simulink model "SBPAMemory"  (R2016a)
settings: Solver=VariableStepAuto  StartTime=0.0  StopTime=1  RelTol=1e-3
values from neighbouring files (symbols this model uses):
  Te = 0.001    [MatlabProjet.m]
libraries: simulink_extras x1
settings Model: Creator=luhernan  LastModifiedBy=luhernan

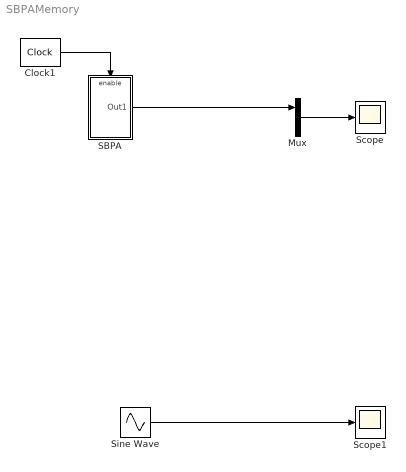
== system SBPAMemory ==
  Clock1 : simulink_extras/Flip Flops/Clock  period=PHorloge
  Mux : Mux  Inputs=2
  SBPA : Subsystem  mask{A=20, Offset=-10}
      mask prompts: A "gain"
  Scope : Scope
  Scope1 : Scope
  Sine Wave : Sin  Amplitude=10  Frequency=6*pi  SampleTime=Te
  wires:
  SBPA/1(Out1) -> Mux/1
  Clock1/1 -> SBPA/Enable
  Sine Wave/1 -> Scope1/1
  Mux/1 -> Scope/1

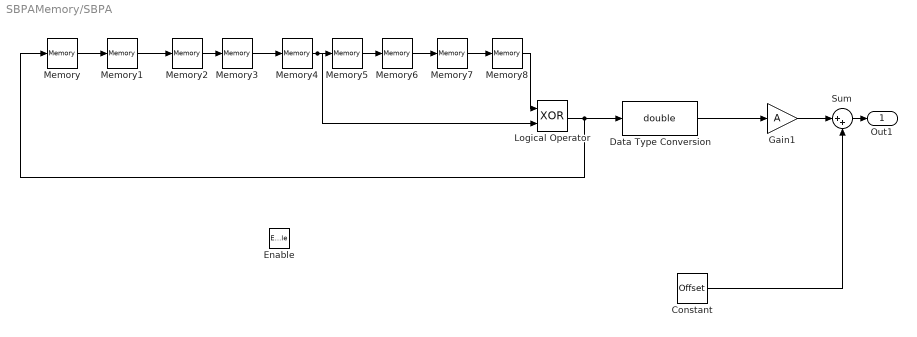
== system SBPAMemory/SBPA ==
  Enable : EnablePort
  Constant : Constant  Value=Offset
  Data Type Conversion : DataTypeConversion  OutMin=[0]  OutMax=[5]  OutDataTypeStr=double
  Gain1 : Gain  Gain=A
  Logical Operator : Logic  Operator=XOR  AllPortsSameDT=off  OutDataTypeStr=boolean
  Memory : Memory  X0=1  InheritSampleTime=on
  Memory{1..8} (8 alike) : Memory  InheritSampleTime=on
  Sum : Sum  Inputs=|++
  Out1 : Outport
  wires:
  Logical Operator/1 -> Memory/1, Data Type Conversion/1
  Memory1/1 -> Memory2/1
  Memory/1 -> Memory1/1
  Memory2/1 -> Memory3/1
  Data Type Conversion/1 -> Gain1/1
  Memory3/1 -> Memory4/1
  Memory4/1 -> Logical Operator/2, Memory5/1
  Memory5/1 -> Memory6/1
  Memory6/1 -> Memory7/1
  Memory7/1 -> Memory8/1
  Memory8/1 -> Logical Operator/1
  Constant/1 -> Sum/2
  Gain1/1 -> Sum/1
  Sum/1 -> Out1/1
